simulink model "Fb_lin_control_stab"  (R2021b)
settings: Solver=ode4  StartTime=0.0  StopTime=20.0  FixedStep=1e-4  RelTol=1e-3
values from neighbouring files (symbols this model uses):
  K = blkdiag(K1, K1, K1, K2)    [Feedback_linearization.m]
settings Model: Creator=pierg  LastModifiedBy=pierg
settings ModelReferenceCC: ModelReferenceMinAlgLoopOccurrences=on

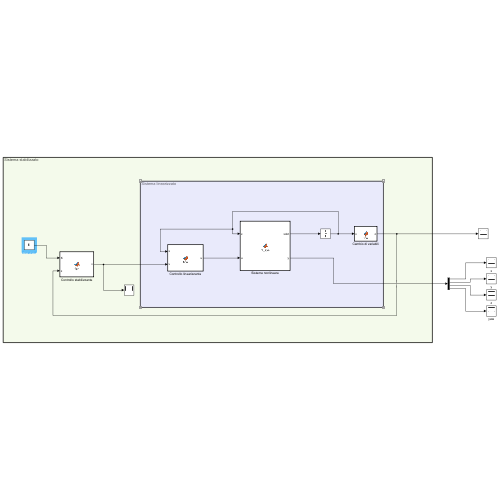
[thumbnail: Simulink's stored preview of the top-level diagram]
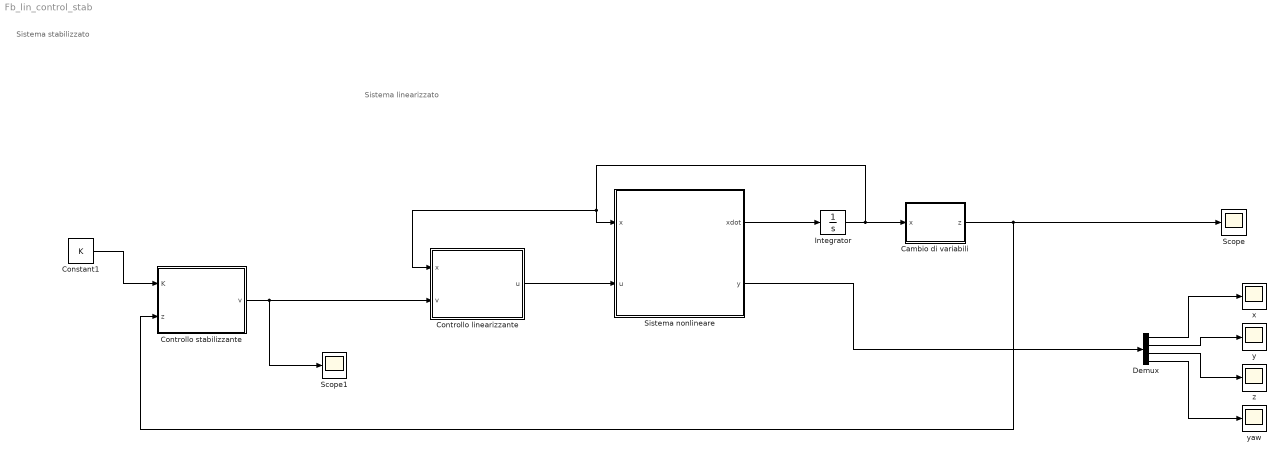
== system Fb_lin_control_stab ==
  note: Sistema stabilizzato
  note: Sistema linearizzato
  Cambio di variabili : MATLAB Function  TreatAsAtomicUnit=on
  Constant1 : Constant  Value=K
  Controllo linearizzante : MATLAB Function  TreatAsAtomicUnit=on
  Controllo stabilizzante : MATLAB Function  TreatAsAtomicUnit=on
  Demux : Demux
  Integrator : Integrator  InitialCondition=[10 5 7 0 0 0 0 0 pi/4 0 0 0 9.81*2 0]'
  Scope : Scope
  Scope1 : Scope
  Sistema nonlineare : MATLAB Function  TreatAsAtomicUnit=on
  x : Scope
  y : Scope
  yaw : Scope
  z : Scope
  wires:
  Sistema nonlineare/1(xdot) -> Integrator/1
  Integrator/1 -> Cambio di variabili/1(x), Controllo linearizzante/1(x), Sistema nonlineare/1(x)
  Controllo linearizzante/1(u) -> Sistema nonlineare/2(u)
  Sistema nonlineare/2(y) -> Demux/1
  Demux/1 -> x/1
  Demux/2 -> y/1
  Demux/3 -> z/1
  Demux/4 -> yaw/1
  Cambio di variabili/1(z) -> Controllo stabilizzante/2(z), Scope/1
  Controllo stabilizzante/1(v) -> Scope1/1, Controllo linearizzante/2(v)
  Constant1/1 -> Controllo stabilizzante/1(K)

== matlab function Fb_lin_control_stab/Sistema nonlineare ==
  data: x input; u input; xdot output; y output
function [xdot, y] = nl_sys(x, u)
% Variabili di stato
x1 = x(1);
x2 = x(2);
x3 = x(3);
x4 = x(4);
x5 = x(5);
x6 = x(6);
x7 = x(7);
x8 = x(8);
x9 = x(9);
x10 = x(10);
x11 = x(11);
x12 = x(12);
u1 = x(13);
du1 = x(14);
% Ingressi di controllo
s1 = u(1);
u2 = u(2);
u3 = u(3);
u4 = u(4);
% Parametri
m = 2; % kg
g = 9.81; % m/s^2
Ix = 1.25; % kg*m^2
Iy = 1.25; % kg*m^2
Iz = 2.5; % kg*m^2
dwx = 0; %m/s^2
dwy = 0; %m/s^2
dwz = 0; %m/s^2

% Il sistema complessivo diventa
f_aa = [x4 x5 x6 -sin(x8)*u1/m sin(x7)*cos(x8)*u1/m -g+cos(x7)*cos(x8)*u1/m x10*cos(x9)-x11*sin(x9) x10*sin(x9)+x11*cos(x9) ...
    x12 0 0 0 du1 0]';
g1_aa = [0 0 0 0 0 0 0 0 0 0 0 0 0 1]';
g2_aa = [0 0 0 0 0 0 0 0 0 1/Ix 0 0 0 0]';
g3_aa = [0 0 0 0 0 0 0 0 0 0 1/Iy 0 0 0]';
g4_aa = [0 0 0 0 0 0 0 0 0 0 0 1/Iz 0 0]';

xdot = f_aa + g1_aa*s1 + g2_aa*u2 + g3_aa*u3 + g4_aa*u4;
y = [x1;x2;x3;x9];

== matlab function Fb_lin_control_stab/Controllo linearizzante ==
  data: x input; u output; v input
function u = fcn(x, v)
% Variabili di stato
x1 = x(1);
x2 = x(2);
x3 = x(3);
x4 = x(4);
x5 = x(5);
x6 = x(6);
x7 = x(7);
x8 = x(8);
x9 = x(9);
x10 = x(10);
x11 = x(11);
x12 = x(12);
u1 = x(13);
du1 = x(14);
% Parametri
m = 2; % kg
g = 9.81; % m/s^2
Ix = 1.25; % kg*m^2
Iy = 1.25; % kg*m^2
Iz = 2.5; % kg*m^2
dwx = 0; %m/s^2
dwy = 0; %m/s^2
dwz = 0; %m/s^2

E = E_fun(Ix,Iy,Iz,m,u1,x7,x8,x9);
Gamma = Gamma_fun(du1,m,u1,x7,x8,x9,x10,x11,x12);

% Controllo necessario alla linearizzazione del modello a valle
u = -inv(E)*Gamma + inv(E)*v;

== matlab function Fb_lin_control_stab/Cambio di variabili ==
  data: x input; z output
function z = fcn(x)
% Variabili di stato
x1 = x(1);
x2 = x(2);
x3 = x(3);
x4 = x(4);
x5 = x(5);
x6 = x(6);
x7 = x(7);
x8 = x(8);
x9 = x(9);
x10 = x(10);
x11 = x(11);
x12 = x(12);
u1 = x(13);
du1 = x(14);
% Parametri
m = 2; % kg
g = 9.81; % m/s^2
Ix = 1.25; % kg*m^2
Iy = 1.25; % kg*m^2
Iz = 2.5; % kg*m^2
dwx = 0; %m/s^2
dwy = 0; %m/s^2
dwz = 0; %m/s^2

z1 = x1; 
z2 = x4; 
z3 = -sin(x8)*u1/m; 
z4 = - (du1*sin(x8))/m - (u1*cos(x8)*(x11*cos(x9) + x10*sin(x9)))/m;  
z5 = x2; 
z6 = x5; 
z7 = sin(x7)*cos(x8)*u1/m; 
z8 = (du1*cos(x8)*sin(x7))/m + (u1*cos(x7)*cos(x8)*(x10*cos(x9) - x11*sin(x9)))/m - (u1*sin(x7)*sin(x8)*(x11*cos(x9) + x10*sin(x9)))/m;
z9 = x3; 
z10 = x6; 
z11 = cos(x7)*cos(x8)*u1/m - g; 
z12 = (du1*cos(x7)*cos(x8))/m - (u1*cos(x7)*sin(x8)*(x11*cos(x9) + x10*sin(x9)))/m - (u1*cos(x8)*sin(x7)*(x10*cos(x9) - x11*sin(x9)))/m;
z13 = x9; 
z14 = x12;

% Nuovo vettore di stato
z = [z1 z2 z3 z4 z5 z6 z7 z8 z9 z10 z11 z12 z13 z14]';

== matlab function Fb_lin_control_stab/Controllo stabilizzante ==
  data: K input; z input; v output
function v = fcn(K, z)
% Controllo stabilizzante
v = -K*z;
